simulink model "PID"  (R2015b)
settings: Solver=ode23t  StartTime=0.0  StopTime=10*360e-6  MaxStep=1e-7  MinStep=1e-9  RelTol=1e-3
undefined symbols (not defined in the file): delay_load, duty_inv, duty_load, Eg, I_ref, Kd1, Ki1, Kp1, l1_val, r_val, rl1_val, t2, T_mach, Vd_val
libraries: powerlib x23, powerlib_meascontrol x2, simulink x1
settings Model: Creator=Akshay  LastModifiedBy=Akshay
settings SolverCC: ZeroCrossAlgorithm=Adaptive
settings DataIOCC: SaveFormat=StructureWithTime
settings HardwareCC: ProdWordSize=32  ProdHWDeviceType=Specified

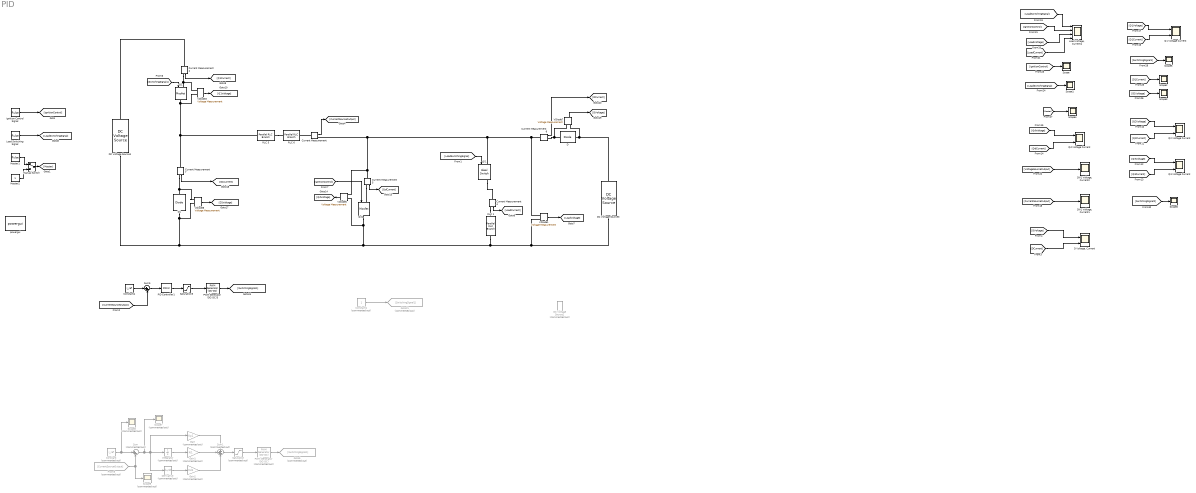
== system PID ==
  " RLC 1" : powerlib/Elements/Parallel RLC Branch  LConnTagsString=a  RConnTagsString=__new0  BranchType=R  Resistance=r_val  Inductance=1e-3  SetiL0=off  InitialCurrent=0  Capacitance=0.1e-6  Setx0=off  InitialVoltage=0  Measurements=None
  " RLC 5" : powerlib/Elements/Parallel RLC Branch  LConnTagsString=a  RConnTagsString=__new0  BranchType=R  Resistance=rl1_val  Inductance=5e-6  SetiL0=off  InitialCurrent=0  Capacitance=0.3e-6  Setx0=off  InitialVoltage=0  Measurements=None
  " RLC 6" : powerlib/Elements/Parallel RLC Branch  LConnTagsString=a  RConnTagsString=__new0  BranchType=L  Resistance=50  Inductance=l1_val  SetiL0=off  InitialCurrent=100  Capacitance=0.3e-6  Setx0=off  InitialVoltage=0  Measurements=None
  Constant : Constant  Commented=on  Value=I_ref
  Constant1 : Constant  Commented=on
  Constant4 : Constant  Value=I_ref
  Current Measurement{,2,4..7} (6 alike) : powerlib/Measurements/Current Measurement  PhasorSimulation=off  OutputType=Complex  PSBequivalent=0
  D : powerlib/Power Electronics/Diode  Ron=0.001  Lon=0  Vf=0.8  IC=0  UseSnubber=off  Rs=500  Cs=250e-9  Measurements=off
  "D Voltage, Current" : Scope  NumInputPorts=2
  D1 : powerlib/Power Electronics/Diode  Ron=0.001  Lon=0  Vf=0.8  IC=0  UseSnubber=off  Rs=500  Cs=250e-9  Measurements=off
  DC Voltage Source1 : powerlib/Electrical Sources/DC Voltage Source  Amplitude=Vd_val  Measurements=Voltage
  DC Voltage Source2 : powerlib/Electrical Sources/DC Voltage Source  Commented=on  Amplitude=Eg  Measurements=Voltage
  DC Voltage Source3 : powerlib/Electrical Sources/DC Voltage Source  Amplitude=80  Measurements=Voltage
  Derivative : Derivative  Commented=on
  From5 : From  Commented=on  GotoTag=CurrentSourceOutput
  Gain : Gain  Commented=on  Gain=Kp1
  Gain1 : Gain  Commented=on  Gain=Ki1
  Gain2 : Gain  Commented=on  Gain=Kd1
  Goto21 : Goto  Commented=on  GotoTag=SwitchingSignal1
  Goto5 : Goto  Commented=on  GotoTag=SwitchingSignal1
  Ignition Control Signal : DiscretePulseGenerator  PulseType=Time based  Period=T_mach  PulseWidth=duty_inv  PhaseDelay=t2-1.8e-6
  Integrator : Integrator  Commented=on
  Load Switching Signal : DiscretePulseGenerator  PulseType=Time based  Period=T_mach  PulseWidth=duty_load  PhaseDelay=delay_load
  "Load Voltage, Current1" : Scope  NumInputPorts=4
  Manual Switch : ManualSwitch
  Master1 : DiscretePulseGenerator  PulseType=Time based  Period=180e-6  PulseWidth=6
  Master2 : Constant
  PID Controller1 : simulink/Continuous/PID Controller  Controller=PID  TimeDomain=Continuous-time  SampleTime=-1  IntegratorMethod=Forward Euler  FilterMethod=Forward Euler  Form=Parallel  UseFilter=on  ControllerParametersSource=internal  P=0.156054293038301  I=15009.4032116143  D=-3.90243468865037e-09  N=39988957.0201293  InitialConditionSource=internal  InitialConditionForIntegrator=0  InitialConditionForFilter=0  ExternalReset=none  LimitOutput=off  UpperSaturationLimit=inf  LowerSaturationLimit=-inf  LinearizeAsGain=on  AntiWindupMode=none  Kb=1  TrackingMode=off  Kt=1  PParamMin=[]  PParamMax=[]  IParamMin=[]  IParamMax=[]  DParamMin=[]  DParamMax=[]  NParamMin=[]  NParamMax=[]  KbParamMin=[]  KbParamMax=[]  KtParamMin=[]  KtParamMax=[]  POutMin=[]  POutMax=[]  IOutMin=[]  IOutMax=[]  DOutMin=[]  DOutMax=[]  NOutMin=[]  NOutMax=[]  KbOutMin=[]  KbOutMax=[]  KtOutMin=[]  KtOutMax=[]  IntegratorOutMin=[]  IntegratorOutMax=[]  FilterOutMin=[]  FilterOutMax=[]  SumOutMin=[]  SumOutMax=[]  SumI1OutMin=[]  SumI1OutMax=[]  SumI2OutMin=[]  SumI2OutMax=[]  SumI3OutMin=[]  SumI3OutMax=[]  SumDOutMin=[]  SumDOutMax=[]  SaturationOutMin=[]  SaturationOutMax=[]  IntegratorContinuousStateAttributes=''  IntegratorStateMustResolveToSignalObject=off  IntegratorRTWStateStorageClass=Auto  FilterContinuousStateAttributes=''  FilterStateMustResolveToSignalObject=off  FilterRTWStateStorageClass=Auto  DifferentiatorICPrevScaledInput=0  DifferentiatorOutMin=[]  DifferentiatorOutMax=[]
  PWM Generator (DC-DC) : powerlib_meascontrol/Pulse & Signal Generators/PWM Generator (DC-DC)  Commented=on  Fsw=5000  Ts=0
  PWM Generator (DC-DC)3 : powerlib_meascontrol/Pulse & Signal Generators/PWM Generator (DC-DC)  Fsw=1000e3  Ts=0
  Q1 : powerlib/Power Electronics/Mosfet  Ron=0.00001  Lon=0  Rd=0.0000000000001  Vfd=0  IC=0  Rs=1e5  Cs=inf  Measurements=off
  Q1 Voltage Current : Scope  NumInputPorts=2
  Q2 Voltage Current : Scope  NumInputPorts=2
  Q3 Voltage Current : Scope  NumInputPorts=2
  Qd Voltage Current : Scope  NumInputPorts=2
  Qd1 : powerlib/Power Electronics/Mosfet  Ron=0.00001  Lon=0  Rd=0.0000000000001  Vfd=0  IC=0  Rs=1e5  Cs=inf  Measurements=off
  Ql1 : powerlib/Power Electronics/Ideal Switch  Ron=0.001  Lon=0  IC=0  Rs=1e5  Cs=inf  Measurements=on
  "SW1 Voltage, Current1" : Scope
  "SW1 Voltage, Current2" : Scope
  Saturation : Saturate  Commented=on  UpperLimit=0.99  LowerLimit=0
  Saturation3 : Saturate  UpperLimit=0.99  LowerLimit=0
  Scope{,1..6} (7 alike) : Scope
  Scope7 : Scope  Commented=on
  Scope8 : Scope  Commented=on
  Scope9 : Scope  Commented=on
  Sum : Sum  Commented=on  Inputs=|+-
  Sum1 : Sum  Commented=on  Inputs=+++
  Sum5 : Sum  Inputs=|+-
  VDiode{1,3,5,7..8} (5 alike) : powerlib/Measurements/Voltage Measurement  PhasorSimulation=off  OutputType=Complex  PSBequivalent=0
  powergui : powerlib/powergui  Priority=1  SimulationMode=Continuous  SolverType=Backward Euler  SampleTime=5e-07  frequency=60  SPID=on  DisableSnubberDevices=off  DisableRonSwitches=off  DisableVfSwitches=off  SwTol=0  DisplayEquations=off  Interpol=off  ExternalGateDelay=off  methode=off  Ts=0  FunctionMessages=off  echomessages=off  HookPort=off  EnableUseOfTLC=off  x0status=zero  frequencyindice=0  Pbase=100e6  ErrMax=1e-4  Iterations=50  UnitsV=kV  UnitsW=MW  buscounter=0  RestoreLinks=warning  ResistiveCurrentMeasurement=off  Frange=[0:2:500]  Ylog=off  Xlog=on  ShowGrid=off  save=off  variable=ZData  structure=ScopeData  ZoomFFT=off  StartTime=0.0  cycles=5  DisplayStyle=2  fundamental=50  FreqAxis=off  MaxFrequency=50000  frequencyindicesteady=1  RmsSteady=1  display=off
  wires:
  Ignition Control Signal/1 -> [IgnitionControl]
  Current Measurement/1 -> [CurrentSourceOutput]
  [SwitchingSignal1] -> Q1/1
  Load Switching Signal/1 -> [LoadSwitchingSignal]
  Manual Switch/1 -> [Master]
  Master1/1 -> Manual Switch/1
  Master2/1 -> Manual Switch/2
  Current Measurement2/1 -> [Q1Current]
  VDiode3/1 -> [Q1Voltage]
  [Q2Voltage] -> Q2 Voltage Current/1
  [Q2Current] -> Q2 Voltage Current/2
  [Q3Voltage] -> Q3 Voltage Current/1
  [Q3Current] -> Q3 Voltage Current/2
  [Q1Voltage] -> Q1 Voltage Current/1
  [Q1Current] -> Q1 Voltage Current/2
  [QdVoltage] -> Qd Voltage Current/1
  [QdCurrent] -> Qd Voltage Current/2
  [LoadSwitchingSignal] -> "Load Voltage, Current1"/1
  [VoltageSourceOutput] -> "SW1 Voltage, Current2"/1
  [IgnitionControl] -> Scope/1
  [LoadSwitchingSignal] -> Scope1/1
  [CurrentSourceOutput] -> "SW1 Voltage, Current1"/1
  Current Measurement7/1 -> [D1Current]
  VDiode8/1 -> [D1Voltage]
  [D1Current] -> Scope2/1
  [D1Voltage] -> Scope3/1
  [Master] -> Scope4/1
  [SwitchingSignal1] -> Scope5/1
  [DVoltage] -> "D Voltage, Current"/1
  [DCurrent] -> "D Voltage, Current"/2
  [SwitchingSignal2] -> Scope6/1
  Constant/1 -> Scope8/1, Sum/1
  From5/1 -> Scope9/1, Sum/2
  Sum/1 -> Scope7/1, Derivative/1, Integrator/1, Gain/1
  Integrator/1 -> Gain1/1
  Derivative/1 -> Gain2/1
  Gain1/1 -> Sum1/2
  Gain/1 -> Sum1/1
  Gain2/1 -> Sum1/3
  Sum1/1 -> Saturation/1
  Saturation/1 -> PWM Generator (DC-DC)/1
  PWM Generator (DC-DC)/1 -> Goto5/1
  Constant1/1 -> Goto21/1
  Sum5/1 -> PID Controller1/1
  Constant4/1 -> Sum5/1
  [CurrentSourceOutput] -> Sum5/2
  PID Controller1/1 -> Saturation3/1
  Saturation3/1 -> PWM Generator (DC-DC)3/1
  PWM Generator (DC-DC)3/1 -> [SwitchingSignal1]
  [LoadVoltage] -> "Load Voltage, Current1"/3
  [LoadCurrent] -> "Load Voltage, Current1"/4
  [IgnitionControl] -> "Load Voltage, Current1"/2
  Current Measurement4/1 -> [LoadCurrent]
  VDiode1/1 -> [LoadVoltage]
  [LoadSwitchingSignal] -> Ql1/1
  [IgnitionControl] -> Qd1/1
  Current Measurement5/1 -> [QdCurrent]
  VDiode5/1 -> [QdVoltage]
  VDiode7/1 -> [DVoltage]
  Current Measurement6/1 -> [DCurrent]
  connections:
  VDiode3/LConn2 -- Q1/RConn1 -- Current Measurement7/LConn1 -- " RLC 5"/LConn1
  Current Measurement2/LConn1 -- DC Voltage Source1/RConn1
  " RLC 5"/RConn1 -- " RLC 6"/LConn1
  Current Measurement/LConn1 -- " RLC 6"/RConn1
  Current Measurement2/RConn1 -- VDiode3/LConn1 -- Q1/LConn1
  Current Measurement7/RConn1 -- D1/RConn1 -- VDiode8/LConn1
  Qd1/RConn1 -- DC Voltage Source1/LConn1 -- VDiode8/LConn2 -- D1/LConn1 -- DC Voltage Source3/LConn1 -- VDiode1/LConn2 -- " RLC 1"/RConn1 -- VDiode5/LConn1
  Current Measurement4/RConn1 -- " RLC 1"/LConn1
  Current Measurement5/LConn1 -- VDiode5/LConn2 -- Current Measurement6/LConn1 -- VDiode1/LConn1 -- Ql1/LConn1 -- Current Measurement/RConn1
  Ql1/RConn1 -- Current Measurement4/LConn1
  Current Measurement5/RConn1 -- Qd1/LConn1
  D/RConn1 -- DC Voltage Source3/RConn1 -- VDiode7/LConn2
  VDiode7/LConn1 -- Current Measurement6/RConn1 -- D/LConn1
